simulink model "smcNL"  (R2022b)
settings: Solver=VariableStepAuto  StartTime=0.0  StopTime=50  RelTol=1e-3
undefined symbols (not defined in the file or in its folder): ang_Lin, d1, d2, DirectCMD, DZ, I, K_hinf, km, MAX_PWM, miu, wb, wcp, wm
libraries: simulink x1
settings Model: Creator=andre  LastModifiedBy=felip
settings SolverCC: AlgebraicLoopSolver=TrustRegion
settings DebuggingCC: UnconnectedInputMsg=warning  UnconnectedOutputMsg=warning  UnconnectedLineMsg=warning  SFMachineParentedDataDiag=warning
settings ModelReferenceCC: EnableRefExpFcnMdlSchedulingChecks=on
settings RTWCC: DLArmComputeVersion=19.05

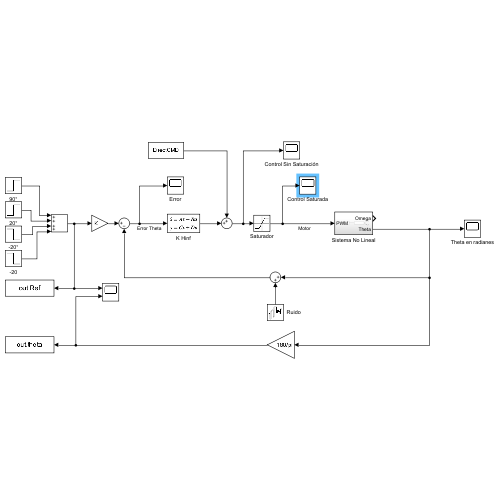
[thumbnail: Simulink's stored preview of the top-level diagram]
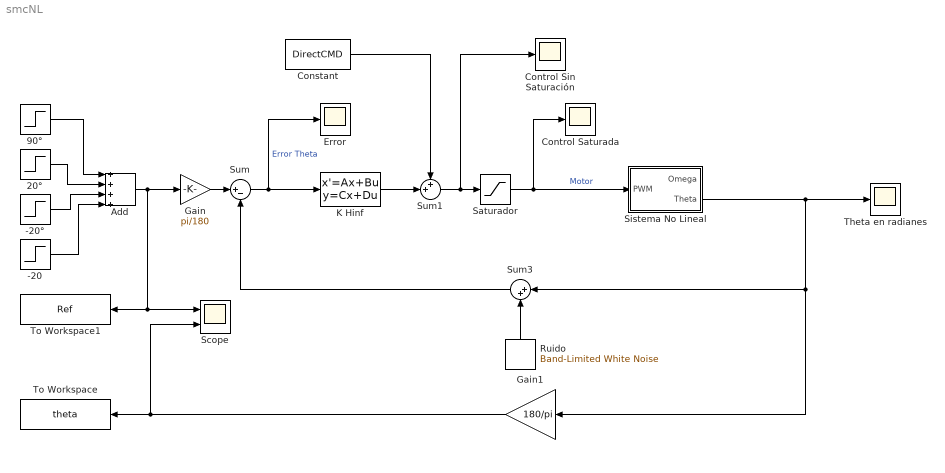
== system smcNL ==
  -20 : Step  Time=30  After=-10  SampleTime=0
  -20° : Step  Time=20  After=-20  SampleTime=0
  20° : Step  Time=10  After=20  SampleTime=0
  90° : Step  Time=0  After=90  SampleTime=0
  Add : Sum  Inputs=++++
  Constant : Constant  Value=DirectCMD
  Control Saturada : Scope
  Control Sin Saturación : Scope
  Error : Scope
  Gain : Gain  Gain=pi/180
  Gain1 : Gain  Gain=180/pi
  K Hinf : StateSpace  A=K_hinf.A  B=K_hinf.B  C=K_hinf.C  D=K_hinf.D  InitialCondition=0
  Ruido : simulink/Sources/Band-Limited White Noise  Cov=[0.001]  Ts=0.1  seed=[23341]
  Saturador : Saturate  UpperLimit=100  LowerLimit=0
  Scope : Scope  NumInputPorts=2
  Sistema No Lineal : Subsystem
  Sum : Sum  Inputs=|+-
  Sum1 : Sum  Inputs=++|
  Sum3 : Sum  Inputs=|++
  Theta en radianes : Scope
  To Workspace : ToWorkspace  VariableName=theta  SaveFormat=Timeseries  SampleTime=-1
  To Workspace1 : ToWorkspace  VariableName=Ref  SaveFormat=Timeseries  SampleTime=-1
  wires:
  Sum/1 -> Error/1, K Hinf/1  "Error Theta"
  90°/1 -> Add/1
  20°/1 -> Add/2
  Sum3/1 -> Sum/2
  Add/1 -> Gain/1, To Workspace1/1, Scope/1
  -20/1 -> Add/4
  Ruido/1 -> Sum3/2
  -20°/1 -> Add/3
  Saturador/1 -> Control Saturada/1, Sistema No Lineal/1(PWM)  "Motor"
  Gain/1 -> Sum/1
  Gain1/1 -> To Workspace/1, Scope/2
  Sistema No Lineal/2(Theta) -> Gain1/1, Sum3/1, Theta en radianes/1
  K Hinf/1 -> Sum1/2
  Sum1/1 -> Control Sin Saturación/1, Saturador/1
  Constant/1 -> Sum1/1

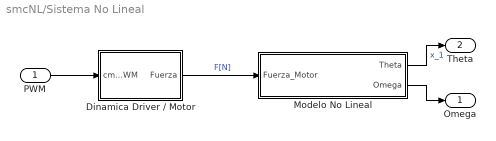
== system smcNL/Sistema No Lineal ==
  PWM : Inport
  Dinamica Driver / Motor : Subsystem
  Modelo No Lineal : Subsystem
  Omega : Outport
  Theta : Outport  Port=2
  wires:
  PWM/1 -> Dinamica Driver / Motor/1(cmd_PWM)
  Dinamica Driver / Motor/1(Fuerza) -> Modelo No Lineal/1(Fuerza_Motor)  "F[N]"
  Modelo No Lineal/1(Theta) -> Theta/1  "x_1"
  Modelo No Lineal/2(Omega) -> Omega/1

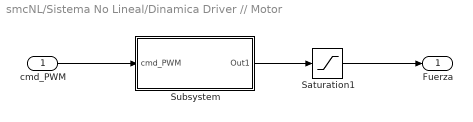
== system smcNL/Sistema No Lineal/Dinamica Driver // Motor ==
  cmd_PWM : Inport
  Saturation1 : Saturate  UpperLimit=MAX_PWM  ZeroCross=off
  Subsystem : Subsystem
  Fuerza : Outport
  wires:
  Saturation1/1 -> Fuerza/1
  cmd_PWM/1 -> Subsystem/1(cmd_PWM)
  Subsystem/1(Out1) -> Saturation1/1

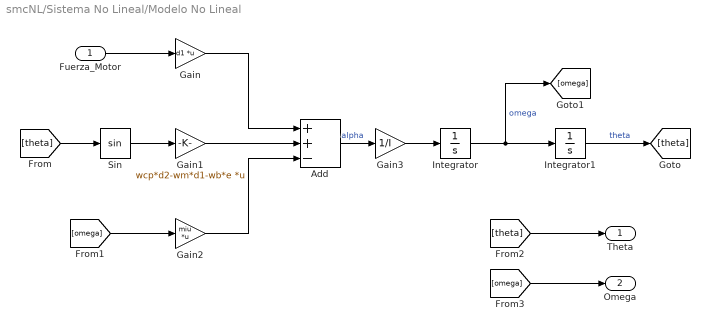
== system smcNL/Sistema No Lineal/Modelo No Lineal ==
  Fuerza_Motor : Inport
  Add : Sum  Inputs=++-
  Gain : Gain  Gain=d1  Multiplication=Matrix(K*u)
  Gain1 : Gain  Gain=wcp*d2-wm*d1-wb*e  Multiplication=Matrix(K*u)
  Gain2 : Gain  Gain=miu  Multiplication=Matrix(K*u)
  Gain3 : Gain  Gain=1/I
  Integrator : Integrator  ZeroCross=off
  Integrator1 : Integrator  InitialCondition=ang_Lin*pi/180  ZeroCross=off
  Sin : Trigonometry
  Theta : Outport
  Omega : Outport  Port=2
  wires:
  [omega] -> Omega/1
  Gain1/1 -> Add/2
  Integrator/1 -> [omega], Integrator1/1  "omega"
  Fuerza_Motor/1 -> Gain/1
  Integrator1/1 -> [theta]  "theta"
  Gain2/1 -> Add/3
  Gain/1 -> Add/1
  Add/1 -> Gain3/1  "alpha"
  [theta] -> Sin/1
  [omega] -> Gain2/1
  [theta] -> Theta/1
  Sin/1 -> Gain1/1
  Gain3/1 -> Integrator/1

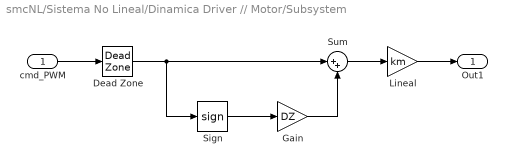
== system smcNL/Sistema No Lineal/Dinamica Driver // Motor/Subsystem ==
  cmd_PWM : Inport
  Dead Zone : DeadZone  LowerValue=-DZ  UpperValue=DZ  ZeroCross=off
  Gain : Gain  Gain=DZ
  Lineal : Gain  Gain=km
  Sign : Signum  ZeroCross=off
  Sum : Sum  Inputs=|++
  Out1 : Outport
  wires:
  cmd_PWM/1 -> Dead Zone/1
  Dead Zone/1 -> Sum/1, Sign/1
  Sum/1 -> Lineal/1
  Sign/1 -> Gain/1
  Gain/1 -> Sum/2
  Lineal/1 -> Out1/1
